simulink model "Pendulo2GDL_RE"  (R2019b)
settings: Solver=ode4  StartTime=0.0  StopTime=10.0  FixedStep=0.01  RelTol=1e-3
values from neighbouring files (symbols this model uses):
  C = [1 0 0 0]    [PenduloDatos.m]
  K = place(Al,Bl,[Pd1 Pd2 Pd3 Pd4])    [PenduloDatos.m]
  K0 = inv(C*(inv(-Al+Bl*K))*Bl)    [PenduloDatos.m]
undefined symbols (not defined in the file or in its folder): Al, Bl
settings Model: Creator=ARQ SEVILLA R  LastModifiedBy=ARQ SEVILLA R

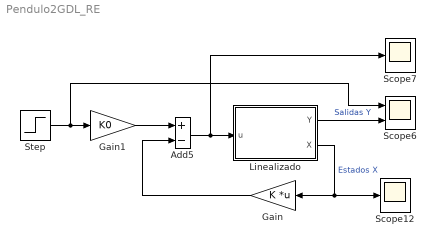
== system Pendulo2GDL_RE ==
  Add5 : Sum  Inputs=+-
  Gain : Gain  Gain=K  Multiplication=Matrix(K*u)
  Gain1 : Gain  Gain=K0
  Linealizado : Subsystem
  Scope12 : Scope
  Scope6 : Scope  NumInputPorts=2
  Scope7 : Scope
  Step : Step  Time=0  After=pi/4  SampleTime=0
  wires:
  Step/1 -> Scope6/1, Gain1/1
  Linealizado/2(X) -> Scope12/1, Gain/1  "Estados X"
  Gain1/1 -> Add5/1
  Gain/1 -> Add5/2
  Linealizado/1(Y) -> Scope6/2  "Salidas Y"
  Add5/1 -> Scope7/1, Linealizado/1(u)

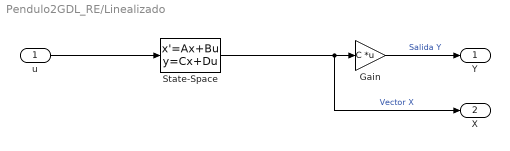
== system Pendulo2GDL_RE/Linealizado ==
  u : Inport
  Gain : Gain  Gain=C  Multiplication=Matrix(K*u)
  State-Space : StateSpace  A=Al  B=Bl  C=eye(4)  D=zeros(4,1)  InitialCondition=[pi/4;0;0;0]
  Y : Outport
  X : Outport  Port=2
  wires:
  State-Space/1 -> X/1, Gain/1  "Vector X"
  Gain/1 -> Y/1  "Salida Y"
  u/1 -> State-Space/1
